simulink model "AMR_DifferentialDrive_24a"  (R2024a)
settings: configuration reference "SharedConfig" (kept outside this file)
undefined symbols (not defined in the file): vehicle_track, vehicle_wheelbase
libraries: simulink_extras x1
settings Model: DataDictionary=configuration_dictionary.sldd  Creator=matlab.cut  LastModifiedBy=matlab.cut
settings ConfigSetRef: SourceName=SharedConfig

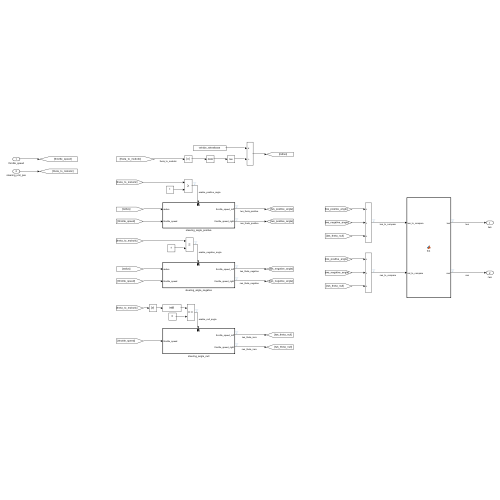
[thumbnail: Simulink's stored preview of the top-level diagram]
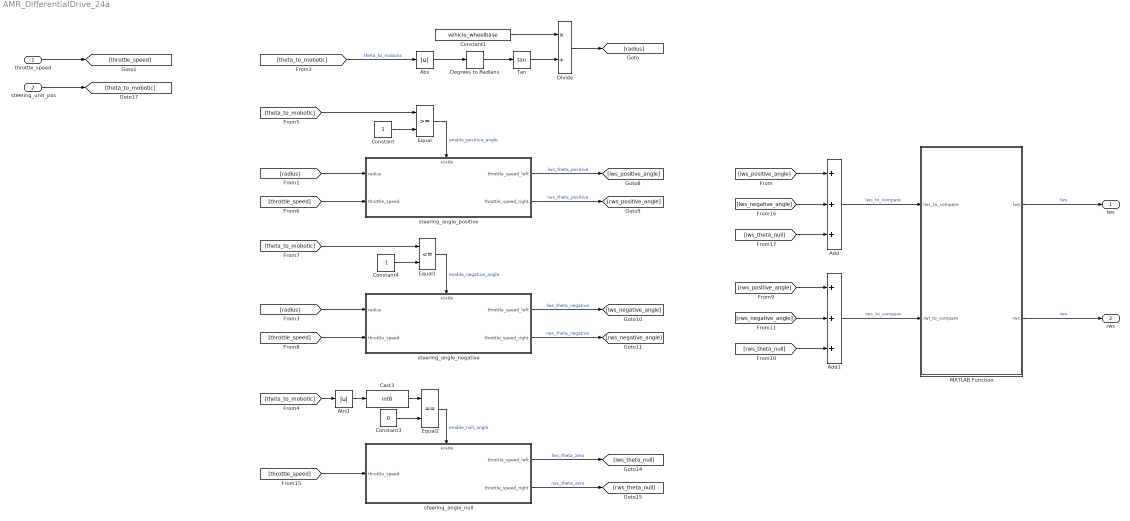
== system AMR_DifferentialDrive_24a ==
  throttle_speed : Inport
  steering_unit_pos : Inport  Port=2
  Abs : Abs  SaturateOnIntegerOverflow=off
  Abs1 : Abs  SaturateOnIntegerOverflow=off
  Add : Sum  Inputs=+++
  Add1 : Sum  Inputs=+++
  Cast3 : DataTypeConversion  OutDataTypeStr=int8  SaturateOnIntegerOverflow=off  RndMeth=Floor
  Constant : Constant
  Constant1 : Constant  Value=vehicle_wheelbase
  Constant3 : Constant  Value=0
  Constant4 : Constant  Value=-1
  Degrees to Radians : simulink_extras/Transformations/Degrees to Radians
  Divide : Product  Inputs=*/
  Equal : RelationalOperator  OutDataTypeStr=boolean  RndMeth=Simplest  InputSameDT=off
  Equal1 : RelationalOperator  Operator=<=  OutDataTypeStr=boolean  RndMeth=Simplest  InputSameDT=off
  Equal2 : RelationalOperator  Operator===  OutDataTypeStr=boolean  RndMeth=Simplest  InputSameDT=off
  MATLAB Function : MATLAB Function  TreatAsAtomicUnit=on
  Tan : Trigonometry  Operator=tan
  steering_angle_negative : Subsystem
  steering_angle_null : Subsystem
  steering_angle_positive : Subsystem
  lws : Outport  OutputWhenDisabled=reset  InitialOutput=[0]
  rws : Outport  Port=2  OutputWhenDisabled=reset  InitialOutput=[0]
  wires:
  MATLAB Function/2(rws) -> rws/1  "rws"
  [throttle_speed] -> steering_angle_negative/2(throttle_speed)
  steering_angle_null/1(throttle_speed_left) -> [lws_theta_null]  "lws_theta_zero"
  Constant4/1 -> Equal1/2
  [lws_negative_angle] -> Add/2
  Abs1/1 -> Cast3/1
  Add/1 -> MATLAB Function/1(lws_to_compare)  "lws_to_compare"
  [lws_positive_angle] -> Add/1
  steering_unit_pos/1 -> [theta_to_mobotic]
  [throttle_speed] -> steering_angle_null/1(throttle_speed)
  [theta_to_mobotic] -> Abs1/1
  [radius] -> steering_angle_negative/1(radius)
  Constant3/1 -> Equal2/2
  [throttle_speed] -> steering_angle_positive/2(throttle_speed)
  Cast3/1 -> Equal2/1
  steering_angle_positive/1(throttle_speed_left) -> [lws_positive_angle]  "lws_theta_positive"
  steering_angle_negative/1(throttle_speed_left) -> [lws_negative_angle]  "lws_theta_negative"
  Equal1/1 -> steering_angle_negative/Enable  "enable_negative_angle"
  [rws_positive_angle] -> Add1/1
  [lws_theta_null] -> Add/3
  [rws_negative_angle] -> Add1/2
  MATLAB Function/1(lws) -> lws/1  "lws"
  Equal2/1 -> steering_angle_null/Enable  "enable_null_angle"
  steering_angle_null/2(throttle_speed_right) -> [rws_theta_null]  "rws_theta_zero"
  Equal/1 -> steering_angle_positive/Enable  "enable_positive_angle"
  Constant/1 -> Equal/2
  steering_angle_positive/2(throttle_speed_right) -> [rws_positive_angle]  "rws_theta_positive"
  [radius] -> steering_angle_positive/1(radius)
  Add1/1 -> MATLAB Function/2(rwl_to_compare)  "rws_to_compare"
  steering_angle_negative/2(throttle_speed_right) -> [rws_negative_angle]  "rws_theta_negative"
  [rws_theta_null] -> Add1/3
  throttle_speed/1 -> [throttle_speed]
  Tan/1 -> Divide/2
  Degrees to Radians/1 -> Tan/1
  [theta_to_mobotic] -> Abs/1  "theta_to_mobotic"
  Abs/1 -> Degrees to Radians/1
  Divide/1 -> [radius]
  Constant1/1 -> Divide/1
  [theta_to_mobotic] -> Equal/1
  [theta_to_mobotic] -> Equal1/1

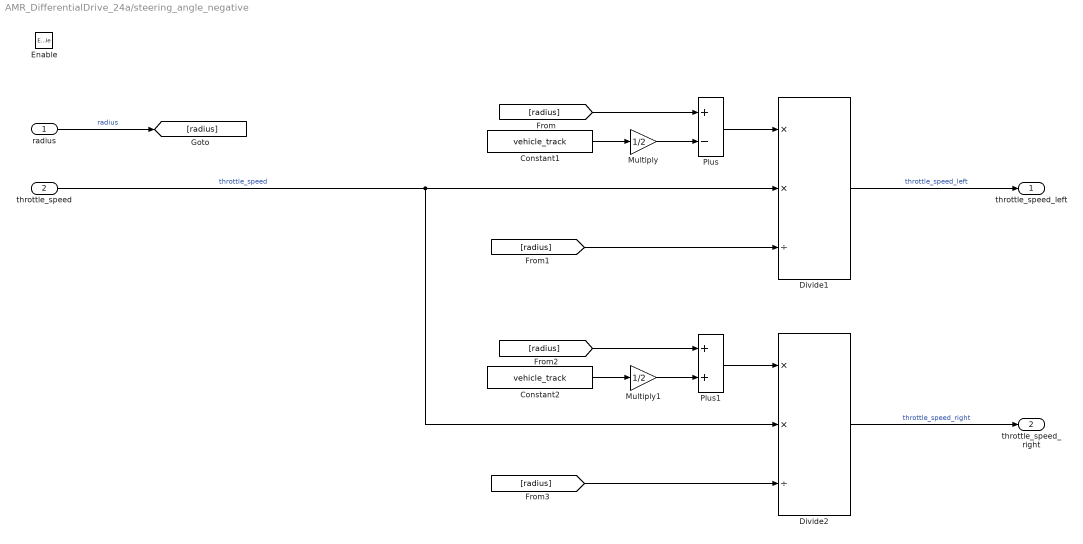
== system AMR_DifferentialDrive_24a/steering_angle_negative ==
  radius : Inport
  throttle_speed : Inport  Port=2
  Enable : EnablePort
  Constant1 : Constant  Value=vehicle_track
  Constant2 : Constant  Value=vehicle_track
  Divide1 : Product  Inputs=**/
  Divide2 : Product  Inputs=**/
  Multiply : Gain  Gain=1/2
  Multiply1 : Gain  Gain=1/2
  Plus : Sum  Inputs=+-
  Plus1 : Sum
  throttle_speed_left : Outport  OutputWhenDisabled=reset  InitialOutput=[0]
  throttle_speed_right : Outport  Port=2  OutputWhenDisabled=reset  InitialOutput=[0]
  wires:
  Multiply/1 -> Plus/2
  Constant2/1 -> Multiply1/1
  Plus1/1 -> Divide2/1
  [radius] -> Divide2/3
  Divide2/1 -> throttle_speed_right/1  "throttle_speed_right"
  throttle_speed/1 -> Divide2/2, Divide1/2  "throttle_speed"
  [radius] -> Divide1/3
  [radius] -> Plus1/1
  Plus/1 -> Divide1/1
  Constant1/1 -> Multiply/1
  [radius] -> Plus/1
  radius/1 -> [radius]  "radius"
  Multiply1/1 -> Plus1/2
  Divide1/1 -> throttle_speed_left/1  "throttle_speed_left"

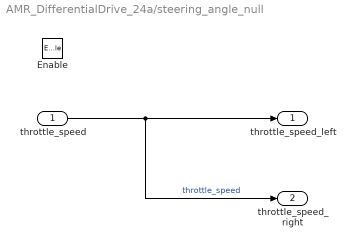
== system AMR_DifferentialDrive_24a/steering_angle_null ==
  throttle_speed : Inport
  Enable : EnablePort
  throttle_speed_left : Outport  OutputWhenDisabled=reset  InitialOutput=[0]
  throttle_speed_right : Outport  Port=2  OutputWhenDisabled=reset  InitialOutput=[0]
  wires:
  throttle_speed/1 -> throttle_speed_right/1, throttle_speed_left/1  "throttle_speed"

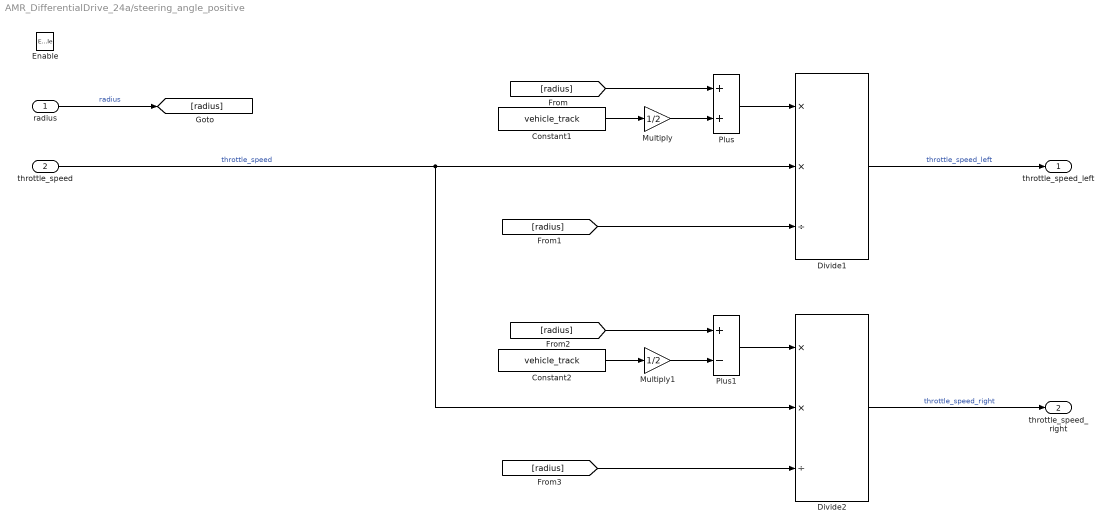
== system AMR_DifferentialDrive_24a/steering_angle_positive ==
  radius : Inport
  throttle_speed : Inport  Port=2
  Enable : EnablePort
  Constant1 : Constant  Value=vehicle_track
  Constant2 : Constant  Value=vehicle_track
  Divide1 : Product  Inputs=**/
  Divide2 : Product  Inputs=**/
  Multiply : Gain  Gain=1/2
  Multiply1 : Gain  Gain=1/2
  Plus : Sum
  Plus1 : Sum  Inputs=+-
  throttle_speed_left : Outport  OutputWhenDisabled=reset  InitialOutput=[0]
  throttle_speed_right : Outport  Port=2  OutputWhenDisabled=reset  InitialOutput=[0]
  wires:
  Constant1/1 -> Multiply/1
  Plus/1 -> Divide1/1
  Divide1/1 -> throttle_speed_left/1  "throttle_speed_left"
  [radius] -> Plus/1
  Multiply/1 -> Plus/2
  [radius] -> Divide1/3
  [radius] -> Divide2/3
  Multiply1/1 -> Plus1/2
  [radius] -> Plus1/1
  Divide2/1 -> throttle_speed_right/1  "throttle_speed_right"
  throttle_speed/1 -> Divide2/2, Divide1/2  "throttle_speed"
  Plus1/1 -> Divide2/1
  Constant2/1 -> Multiply1/1
  radius/1 -> [radius]  "radius"

== matlab function AMR_DifferentialDrive_24a/MATLAB Function ==
  data: lws_to_compare input; lws output; rwl_to_compare input; rws output
function [lws, rws] = fcn(lws_to_compare, rwl_to_compare)

max_curtis_speed = 3000; % rpm

if abs(lws_to_compare) >= max_curtis_speed
    rws = rwl_to_compare * (max_curtis_speed / abs(lws_to_compare));
    lws = sign(lws_to_compare) * max_curtis_speed;
elseif abs(rwl_to_compare) >= max_curtis_speed
    lws = lws_to_compare * (max_curtis_speed / abs(rwl_to_compare));
    rws = sign(rwl_to_compare) * max_curtis_speed;
else
    lws = lws_to_compare;
    rws = rwl_to_compare;
end
